simulink model "hydroelectric"  (R2019a)
settings: Solver=VariableStepAuto  StartTime=0.0  StopTime=0.1  RelTol=1e-3
libraries: powerlib x7, sps_avr x1, powerlib_meascontrol x1, dspstat3 x1
settings Model: Creator=Nazhan  LastModifiedBy=Nazhan

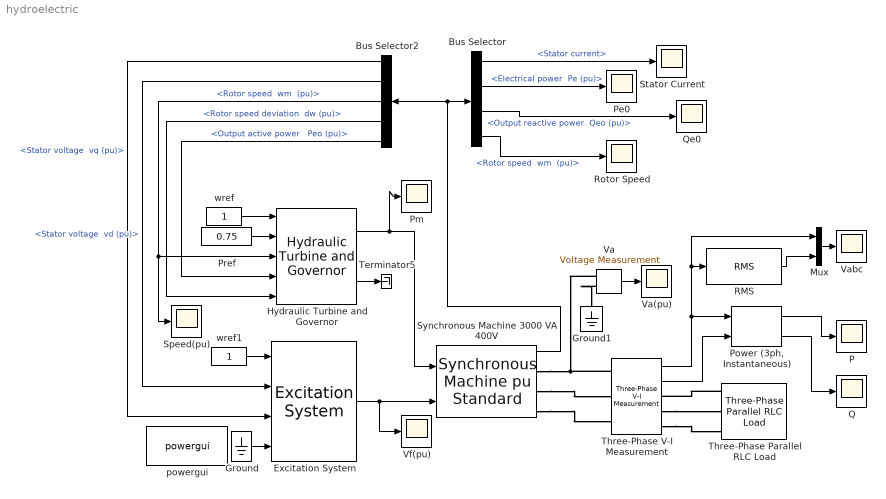
== system hydroelectric ==
  Bus Selector : BusSelector  OutputSignals="Stator current,Mechanical.Electrical power  Pe (pu),Output reactive power  Qeo (pu),Mechanical.Rotor speed  wm  (pu)"
  Bus Selector2 : BusSelector  OutputSignals="dq0 components.Stator voltage  vq (pu),dq0 components.Stator voltage  vd (pu),Mechanical.Rotor speed  wm  (pu),Mechanical.Rotor speed deviation  dw (pu),Output active power   Peo (pu)"
  Excitation System : sps_avr/Excitation System  tr=20e-3  reg=[ 300, 0.001 ]  exc=[ 1, 0 ]  tgr=[ 0, 0 ]  damp=[ 0.001, 0.1 ]  sat=[ 0, 0 ]  lim=[ -11.5, 11.5, 0 ]  v0="[1.0  1.28]"
      settings: SourceProductName=Simscape Electrical  SourceProductBaseCode=PS
  Ground : Ground
  Ground1 : powerlib/Elements/Ground  LConnTagsString=a
      settings: SourceProductName=Simscape Electrical
  Hydraulic Turbine and Governor : powerlib/Machines/Hydraulic Turbine and Governor  sm="[ 10/3  0.07 ]"  gate="[  0.01  0.97518  -0.1  0.1 ]"  reg="[  0.05  1.163  0.105  0  0.01  ]"  hyd="[  0  2.67  ]"  dref=0  po=0.7516
      settings: SourceProductName=Simscape Electrical  SourceProductBaseCode=PS
  Mux : Mux  Inputs=2
  P : Scope
  Pe0 : Scope
  Pm : Scope
  "Power (3ph, Instantaneous)" : powerlib_meascontrol/Measurements/Power (3ph, Instantaneous)
      settings: SourceProductName=Simscape Electrical
  Pref : Constant  Value=0.75
  Q : Scope
  Qe0 : Scope
  RMS : dspstat3/RMS  run=off  directionMode=Each column  dimension=1  InputProcessing=Columns as channels (frame based)  reset_popup=None
  Rotor Speed : Scope
  Speed(pu) : Scope
  Stator Current : Scope
  Synchronous Machine 3000 VA 400V : powerlib/Machines/Synchronous Machine pu Standard  PresetModel=No  MechanicalLoad=Mechanical power Pm  ShowDetailedParameters=on  RotorType=Salient-pole  Units=per unit standard parameters  MeasurementBus=off  NominalParameters="[ 3000  400   60 ]"  Reactances1=[ 31 32 33 34 35 36 37 ]  Reactances2=[ 1.305, 0.296, 0.252, 0.474, 0.243, 0.18 ]  dAxisTimeConstants=Short-circuit  qAxisTimeConstants=Open-circuit  TimeConstants1=[]  TimeConstants2=[]  TimeConstants3=[]  TimeConstants4=[]  TimeConstants5=[ 1.01, 0.053, 0.1 ]  TimeConstants6=[]  TimeConstants7=[]  TimeConstants8=[]  StatorResistance=2.8544e-3  Mechanical=[ 3.2 0 2]  PolePairs=2  InitialConditions=[0 -94.2826 0.750185 0.750185 0.750185 -24.943 -144.943 95.057 1.29071]  SetSaturation=off  Saturation=[0.6404,0.7127,0.8441,0.9214,0.9956,1.082,1.19,1.316,1.457;0.7,0.7698,0.8872,0.9466,0.9969,1.046,1.1,1.151,1.201]  LoadFlowParameters=[1 150000000 0 0]  TsPowergui=0  TsBlock=-1  IterativeModel=Trapezoidal non iterative  IterativeDiscreteModel=Trapezoidal non iterative  BusType=PV  Pref=1800  Qref=0  Qmin=-Inf  Qmax=Inf  PLF=0  QLF=0
      settings: AttributesFormatString=\n\n  SourceProductName=Simscape Electrical
  Terminator5 : Terminator
  Three-Phase Parallel RLC Load : powerlib/Elements/Three-Phase Parallel RLC Load  LConnTagsString=A|B|C  Configuration=Y (grounded)  NominalVoltage=1000  Vabc=[1e3 1e3 1e3]  Vabcp=[1e3 1e3 1e3]  NominalFrequency=60  UnbalancedPower=off  ActivePower=10e3  InductivePower=100  CapacitivePower=100  Pabc=[10e3 9e3 11e3]  QLabc=[100 90 110]  QCabc=[100 90 110]  Pabcp=[10e3 9e3 11e3]  QLabcp=[100 90 110]  QCabcp=[100 90 110]  Measurements=None  LoadType=constant Z
      settings: SourceProductName=Simscape Electrical
  Three-Phase V-I Measurement : powerlib/Measurements/Three-Phase V-I Measurement  VoltageMeasurement=phase-to-ground  SetLabelV=off  LabelV=Vabc  Vpu=off  VpuLL=off  CurrentMeasurement=yes  SetLabelI=off  LabelI=Iabc  Ipu=off  Pbase=100e6  Vbase=500e3  OutputType=Complex  PhasorSimulation=off  PSBequivalent=0
      settings: SourceProductName=Simscape Electrical
  Va : powerlib/Measurements/Voltage Measurement  Tag=PoWeRsYsTeMmEaSuReMeNt  PhasorSimulation=off  OutputType=Magnitude  PSBequivalent=0
      settings: SourceProductName=Simscape Electrical
  Va(pu) : Scope
  Vabc : Scope
  Vf(pu) : Scope
  powergui : powerlib/powergui  Priority=1  SimulationMode=Continuous  SampleTime=50e-6  frequency=60  Iterations=50  frequencyindice=60  Pbase=100e6  ErrMax=1e-4  UnitsV=kV  UnitsW=MW  buscounter=0  FunctionMessages=off  echomessages=off  EnableUseOfTLC=off  CurrentSourceSwitches=off  DisableSnubberDevices=off  DisableRonSwitches=off  DisableVfSwitches=off  DisplayEquations=off  AutomaticDiscreteSolvers=off  SolverType=Tustin/Backward Euler (TBE)  Interpol=off  ExternalGateDelay=off  methode=off  Ts=100  x0status=blocks  SPID=on  SwTol=0  HookPort=off  NonlinearTolerance=0  nMaxIteration=15  ContinueOnMaxIteration=off  RestoreLinks=warning  ResistiveCurrentMeasurement=off  Frange=[0:2:500]  Ylog=off  Xlog=on  ShowGrid=off  save=off  variable=ZData  structure=0  ZoomFFT=off  StartTime=0.0  cycles=1  DisplayStyle=1  fundamental=60  FreqAxis=off  MaxFrequency=1000  frequencyindicesteady=1  RmsSteady=1  display=off
      settings: SourceProductName=Simscape Electrical
  wref : Constant
  wref1 : Constant
  wires:
  Excitation System/1 -> Synchronous Machine 3000 VA 400V/2, Vf(pu)/1
  Hydraulic Turbine and Governor/2 -> Terminator5/1
  Hydraulic Turbine and Governor/1 -> Synchronous Machine 3000 VA 400V/1, Pm/1
  Ground/1 -> Excitation System/4
  wref/1 -> Hydraulic Turbine and Governor/1
  Pref/1 -> Hydraulic Turbine and Governor/2
  Bus Selector2/5 -> Hydraulic Turbine and Governor/4  "<Output active power   Peo (pu)>"
  Bus Selector2/4 -> Hydraulic Turbine and Governor/5  "<Rotor speed deviation  dw (pu)>"
  Bus Selector2/3 -> Speed(pu)/1, Hydraulic Turbine and Governor/3  "<Rotor speed  wm  (pu)>"
  Bus Selector2/2 -> Excitation System/2  "<Stator voltage  vd (pu)>"
  Bus Selector2/1 -> Excitation System/3  "<Stator voltage  vq (pu)>"
  wref1/1 -> Excitation System/1
  Synchronous Machine 3000 VA 400V/1 -> Bus Selector2/1, Bus Selector/1
  Three-Phase V-I Measurement/1 -> RMS/1, Mux/1, "Power (3ph, Instantaneous)"/1
  Three-Phase V-I Measurement/2 -> "Power (3ph, Instantaneous)"/2
  RMS/1 -> Mux/2
  Bus Selector/1 -> Stator Current/1  "<Stator current>"
  Bus Selector/2 -> Pe0/1  "<Electrical power  Pe (pu)>"
  Bus Selector/3 -> Qe0/1  "<Output reactive power  Qeo (pu)>"
  Va/1 -> Va(pu)/1
  "Power (3ph, Instantaneous)"/1 -> P/1
  "Power (3ph, Instantaneous)"/2 -> Q/1
  Mux/1 -> Vabc/1
  Bus Selector/4 -> Rotor Speed/1  "<Rotor speed  wm  (pu)>"
  connections:
  Three-Phase V-I Measurement/LConn1 -- Synchronous Machine 3000 VA 400V/RConn1 -- Va/LConn1
  Synchronous Machine 3000 VA 400V/RConn2 -- Three-Phase V-I Measurement/LConn2
  Synchronous Machine 3000 VA 400V/RConn3 -- Three-Phase V-I Measurement/LConn3
  Three-Phase Parallel RLC Load/LConn1 -- Three-Phase V-I Measurement/RConn1
  Three-Phase V-I Measurement/RConn2 -- Three-Phase Parallel RLC Load/LConn2
  Three-Phase V-I Measurement/RConn3 -- Three-Phase Parallel RLC Load/LConn3
  Va/LConn2 -- Ground1/LConn1
